simulink model "Motor_Position_Modelw_friction_6_closed_loop_ImplementLead"  (R2018b)
settings: Solver=ode45  StartTime=0.0  StopTime=0.4  FixedStep=.0001  RelTol=1e-6  AbsTol=1e-6  EnableMultiTasking=on
values from neighbouring files (symbols this model uses):
  Fo = 1    [Motor_Position_Modelw_friction_6m_Lab.m]
  Gain = 23    [Motor_Position_Modelw_friction_6m_Lab.m]
  Kinetic_friction_transition_rate = 1000    [Motor_Position_Modelw_friction_6m_Lab.m]
  Omegan = 2*pi*frequency_n    (= 50)    [Motor_Position_Modelw_friction_6m_Lab.m]
  Zeta = 0.74    [Motor_Position_Modelw_friction_6m_Lab.m]
settings Model: Creator=davet  LastModifiedBy=luonc
settings SolverCC: AutoScaleAbsTol=off
settings DataIOCC: LimitDataPoints=on  SaveFormat=Array  SignalLoggingSaveFormat=ModelDataLogs  SignalLoggingName=sigsOut
settings OptimizationCC: BlockReduction=off  BooleanDataType=off  ExpressionDepthLimit=2147483647  LifeSpan=inf
settings DebuggingCC: SaveWithParameterizedLinksMsg=none  UnderspecifiedInitializationDetection=Classic  MergeDetectMultiDrivingBlocksExec=none  SignalResolutionControl=TryResolveAllWithWarning  MultiTaskDSMMsg=warning  MultiTaskCondExecSysMsg=none  FcnCallInpInsideContextMsg=warning  StateNameClashWarn=warning  SFUnexpectedBacktrackingDiag=warning  SFNoUnconditionalDefaultTransitionDiag=warning  SFExecutionAtInitializationDiag=none
settings HardwareCC: ProdBitPerPointer=32  ProdBitPerSizeT=32  ProdBitPerPtrDiffT=32  ProdLargestAtomicFloat=None  ProdIntDivRoundTo=Undefined  ProdEndianess=Unspecified  ProdWordSize=32  ProdHWDeviceType=32-bit Generic  TargetUnknown=on
settings ModelReferenceCC: PropagateSignalLabelsOutOfModel=off
settings SFSimCC: SimUseLocalCustomCode=off
settings RTWCC: RTWUseLocalCustomCode=off
settings CodeAppCC: StateflowObjectComments=on
settings GRTTargetCC: TargetLangStandard=C89/C90 (ANSI)  ModelReferenceCompliant=off  ParMdlRefBuildCompliant=off  CompOptLevelCompliant=off  ConcurrentExecutionCompliant=off  GeneratePreprocessorConditionals=Disable all  CombineOutputUpdateFcns=off  MatFileLogging=off  GRTInterface=on
settings ConfigComp: CovMetricSettings=dw  CovHtmlReporting=on  CovSaveCumulativeToWorkspaceVar=on  CovSaveSingleToWorkspaceVar=on  CovExternalEMLEnable=off

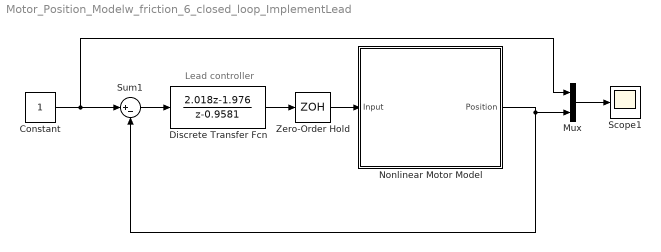
== system Motor_Position_Modelw_friction_6_closed_loop_ImplementLead ==
  note: Lead controller
  Constant : Constant
  Discrete Transfer Fcn : DiscreteTransferFcn  Numerator=[2.018 -1.976]  Denominator=[1 -0.9581]  SampleTime=0.001
  Mux : Mux  Inputs=2
  Nonlinear Motor Model : Subsystem
  Scope1 : Scope
  Sum1 : Sum  Inputs=|+-  SaturateOnIntegerOverflow=on  InputSameDT=on  OutDataTypeStr=Inherit: Same as first input
  Zero-Order Hold : ZeroOrderHold  SampleTime=0.001
  wires:
  Sum1/1 -> Discrete Transfer Fcn/1
  Constant/1 -> Mux/1, Sum1/1
  Nonlinear Motor Model/1(Position) -> Mux/2, Sum1/2
  Mux/1 -> Scope1/1
  Discrete Transfer Fcn/1 -> Zero-Order Hold/1
  Zero-Order Hold/1 -> Nonlinear Motor Model/1(Input)

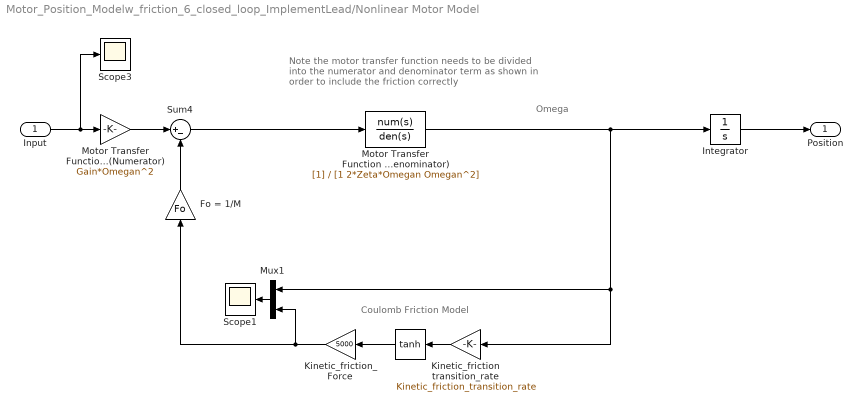
== system Motor_Position_Modelw_friction_6_closed_loop_ImplementLead/Nonlinear Motor Model ==
  note: Omega
  note: Coulomb Friction Model
  note: Note the motor transfer function needs to be divided
      |  into the numerator and denominator term as shown
      | in order to include the friction correctly
  Input : Inport
  " " : Trigonometry  Operator=tanh
  Fo = 1/M : Gain  Gain=Fo  SaturateOnIntegerOverflow=on  OutDataTypeStr=Inherit: Same as input  ParamDataTypeStr=Inherit: Same as input
  Integrator : Integrator
  Kinetic_friction transition_rate : Gain  Gain=Kinetic_friction_transition_rate
  Kinetic_friction_Force : Gain  Gain=5000
  Motor Transfer Function (Numerator) : Gain  Gain=Gain*Omegan^2  SaturateOnIntegerOverflow=on  OutDataTypeStr=Inherit: Same as input  ParamDataTypeStr=Inherit: Same as input
  Motor Transfer Function (Denominator) : TransferFcn  Denominator=[1 2*Zeta*Omegan Omegan^2]
  Mux1 : Mux  Inputs=2
  Scope1 : Scope
  Scope3 : Scope
  Sum4 : Sum  Inputs=|+-  SaturateOnIntegerOverflow=on  InputSameDT=on  OutDataTypeStr=Inherit: Same as first input
  Position : Outport
  wires:
  Motor Transfer Function (Denominator)/1 -> Integrator/1, Kinetic_friction transition_rate/1, Mux1/1
  Input/1 -> Scope3/1, Motor Transfer Function (Numerator)/1
  " "/1 -> Kinetic_friction_Force/1
  Kinetic_friction transition_rate/1 -> " "/1
  Kinetic_friction_Force/1 -> Mux1/2, Fo = 1/M/1
  Mux1/1 -> Scope1/1
  Fo = 1/M/1 -> Sum4/2
  Sum4/1 -> Motor Transfer Function (Denominator)/1
  Motor Transfer Function (Numerator)/1 -> Sum4/1
  Integrator/1 -> Position/1
